simulink model "publish_mqtt"  (R2025b)
settings: Solver=FixedStepDiscrete  StartTime=0.0  StopTime=100  FixedStep=1  RelTol=1e-3
InitFcn:
  | % 1. Définition du vecteur temps (100 secondes)
  | t = (0:100)';
  | 
  | % 2. Génération des données de base (Normales)
  | temp_data = -70 + randn(length(t), 1) * 0.1;
  | gforce_data = 1.0 + randn(length(t), 1) * 0.02;
  | 
  | % 3. Génération de 3 instants aléatoires pour les chocs
  | % On choisit 3 nombres uniques entre 10 et 90 secondes
  | instants_chocs = randperm(80, 3) + 10;
  | 
  | % 4. Injection des anomalies aux instants tirés au sort
  | for i = 1:3
  |     idx = instants_chocs(i);
  |     % Un choc physique aléatoire entre 4.0 et 8.0 G
  |     gforce_data(idx) = 4.0 + rand() * 4.0;
  | 
  |     % Une hausse de température consécutive au choc (durée 5 secondes)
  |     fin_hausse = min(idx + 5, length(t));
  |     temp_data(idx:fin_hausse) = temp_data(idx:fin_hausse) + (5.0 + rand() * 10.0);
  | end
  | 
  | % 5. Forcer l'envoi des variables dans le Workspace principal de MATLAB
  | assignin('base', 'sim_temp', timeseries(temp_data, t));
  | assignin('base', 'sim_gforce', timeseries(gforce_data, t));
  | 
  | % Petit message de confirmation dans la console
  | disp(['[Simulink] Dataset généré. Chocs injectés aux secondes : ', num2str(sort(instants_chocs))]);
settings Model: Creator=mehdi  LastModifiedBy=mehdi

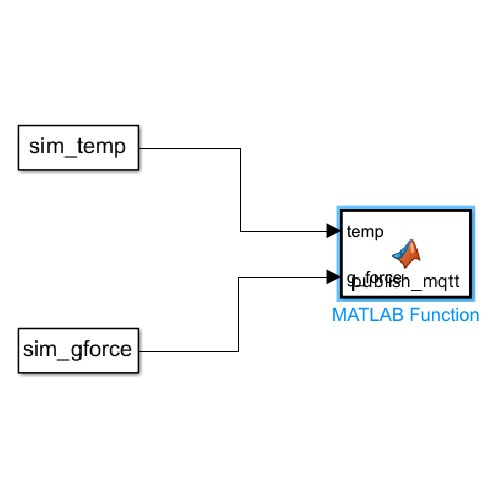
[thumbnail: Simulink's stored preview of the top-level diagram]
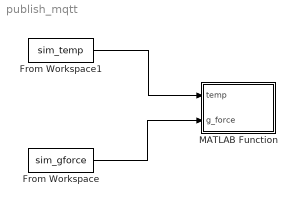
== system publish_mqtt ==
  From Workspace : FromWorkspace  VariableName=sim_gforce
  From Workspace1 : FromWorkspace  VariableName=sim_temp
  MATLAB Function : MATLAB Function  TreatAsAtomicUnit=on
  wires:
  From Workspace1/1 -> MATLAB Function/1(temp)
  From Workspace/1 -> MATLAB Function/2(g_force)

== matlab function publish_mqtt/MATLAB Function ==
  data: temp input; g_force input
function publish_mqtt(temp, g_force)
    coder.extrinsic('system', 'num2str');
    
    t_str = num2str(temp);
    g_str = num2str(g_force);
    
    python_exe = 'C:\Users\mehdi\anaconda3\python.exe';
    script_path = 'C:\Users\mehdi\ThermoPath\src\simulink_bridge.py';
    
    cmd = [python_exe, ' ', script_path, ' ', t_str, ' ', g_str];
    
    system(cmd);
end
